simulink model "ode_engine_sim - preorg backup"  (R2022a)
settings: Solver=VariableStepAuto  StartTime=0.0  StopTime=10.0  RelTol=1e-3
model workspace (MAT data in the model file):
  A_inj = 1
  A_throat = 1
  C_d = 0.7
  L = 1
  L_grain = 1
  TCrit = 309.57
  V_tank = 1
  a = 1
  m_reg = 1
  n = 1
  rhoCrit = 452
  rho_f = 1
settings Model: Creator=Artem Sotnikov  LastModifiedBy=Artem Sotnikov

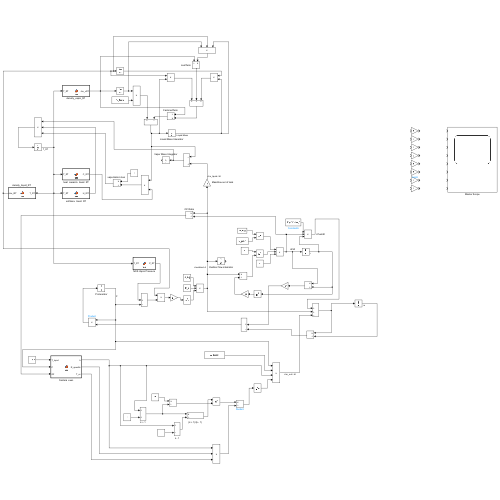
[thumbnail: Simulink's stored preview of the top-level diagram]
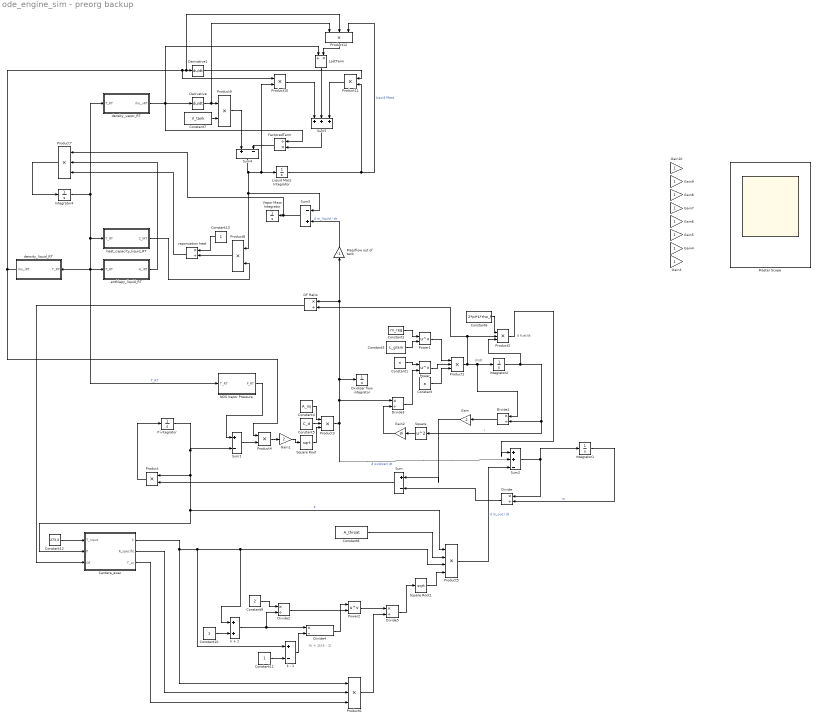
== system ode_engine_sim - preorg backup ==
  note: (k + 1)/(k - 1)
  note: d fuel/dt
  note: dr/dt
  Cantera_exec : MATLAB Function  TreatAsAtomicUnit=on
  Constant : Constant  Value=a
  Constant1 : Constant  Value=n
  Constant10 : Constant
  Constant11 : Constant
  Constant12 : Constant  Value=273.3
  Constant13 : Constant
  Constant2 : Constant  Value=m_reg
  Constant3 : Constant  Value=L_grain
  Constant4 : Constant  Value=A_inj
  Constant5 : Constant  Value=C_d
  Constant6 : Constant  Value=2*pi*L*rho_f
  Constant7 : Constant  Value=V_tank
  Constant8 : Constant  Value=A_throat
  Constant9 : Constant  Value=2
  Derivative : Derivative
  Derivative1 : Derivative
  Divide{,1..5} (6 alike) : Product  Inputs=*/
  FactoredTerm : Product  Inputs=/*
  Gain : Gain  Gain=2
  Gain1 : Gain  Gain=2
  Gain{3..10} (8 alike) : Gain
  Gain2 : Gain  Gain=pi
  Integrator1 : Integrator
  Integrator2 : Integrator
  Integrator4 : Integrator
  LastTerm : Product  Inputs=/*
  Liquid Mass Integrator : Integrator
  Massflow out of tank : Gain  Gain=-1
  Master Scope : Scope  NumInputPorts=8
  NOS Vapor Pressure : MATLAB Function  TreatAsAtomicUnit=on
  OF Ratio : Product  Inputs=*/
  Oxidizer flow integrator : Integrator
  P integrator : Integrator
  Power : Math  Operator=pow
  Power1 : Math  Operator=pow
  Power2 : Math  Operator=pow
  Product{,4,8..11} (6 alike) : Product
  Product{1..3,6..7,12} (6 alike) : Product  Inputs=3
  Product5 : Product  Inputs=4
  Square : Math  Operator=square
  Square Root : Sqrt
  Square Root1 : Sqrt
  Sum : Sum  Inputs=|+-
  Sum1 : Sum  Inputs=|+-
  Sum2 : Sum  Inputs=|++-
  Sum3 : Sum  Inputs=-+
  Sum4 : Sum  Inputs=+-
  Sum5 : Sum  Inputs=+++
  Vapor Mass Integrator : Integrator
  "density_liquid_RT " : MATLAB Function  TreatAsAtomicUnit=on
  density_vapor_RT : MATLAB Function  TreatAsAtomicUnit=on
  enthlapy_liquid_RT : MATLAB Function  TreatAsAtomicUnit=on
  heat_capacity_liquid_RT : MATLAB Function  TreatAsAtomicUnit=on
  k + 1 : Sum
  k - 1 : Sum  Inputs=+-
  vaporization heat : Product  Inputs=*/
  wires:
  P integrator/1 -> Sum1/2, Product/1, Product5/1, Cantera_exec/2(P)  "P"
  Sum/1 -> Product/2
  Integrator1/1 -> Divide/2  "m"
  Product/1 -> P integrator/1
  Sum2/1 -> Integrator1/1, Divide/1
  Divide/1 -> Sum/2
  Product1/1 -> Integrator2/1, Divide1/1, Product2/2, OF Ratio/2
  Integrator2/1 -> Product2/3, Divide1/2, Square/1  "r"
  Divide1/1 -> Gain/1
  Gain/1 -> Sum/1
  Power/1 -> Product1/2
  Power1/1 -> Product1/1
  Constant/1 -> Product1/3
  Constant1/1 -> Power/1
  Constant2/1 -> Power1/1
  Constant3/1 -> Power1/2
  Divide3/1 -> Power/2
  Constant5/1 -> Product3/2
  Constant4/1 -> Product3/1
  Square Root/1 -> Product3/3
  Product3/1 -> Sum2/2, Divide3/1, Massflow out of tank/1, OF Ratio/1, Oxidizer flow integrator/1  "d oxidizer/ dt"
  Gain1/1 -> Square Root/1
  NOS Vapor Pressure/1(P_RT) -> Sum1/1
  Product4/1 -> Gain1/1
  Sum1/1 -> Product4/2
  "density_liquid_RT "/1(rho_lRT) -> Product10/1, Product12/2, Derivative1/1, Product4/1
  Square/1 -> Gain2/1
  Gain2/1 -> Divide3/2
  Product2/1 -> Sum2/1
  Constant6/1 -> Product2/1
  Product5/1 -> Sum2/3  "d m_out / dt"
  Square Root1/1 -> Product5/4
  Constant8/1 -> Product5/2
  Cantera_exec/1(k) -> Product6/1, Product5/3, k + 1/1, k - 1/1
  Constant9/1 -> Divide2/1
  Constant10/1 -> k + 1/2
  k + 1/1 -> Divide4/1, Divide2/2
  k - 1/1 -> Divide4/2
  Constant11/1 -> k - 1/2
  Divide4/1 -> Power2/1
  Divide2/1 -> Power2/2
  Product6/1 -> Divide5/2
  Power2/1 -> Divide5/1
  Cantera_exec/2(R_specific) -> Product6/2
  Constant12/1 -> Cantera_exec/1(T_input)
  OF Ratio/1 -> Cantera_exec/3(OF)
  Cantera_exec/3(T_cc) -> Product6/3
  Divide5/1 -> Square Root1/1
  Integrator4/1 -> NOS Vapor Pressure/1(T_RT), "density_liquid_RT "/1(T_RT), enthlapy_liquid_RT/1(T_RT), heat_capacity_liquid_RT/1(T_RT), density_vapor_RT/1(T_RT)  "T_RT"
  Product7/1 -> Integrator4/1
  enthlapy_liquid_RT/1(H_lRT) -> Product7/2
  Constant13/1 -> vaporization heat/1
  Product8/1 -> vaporization heat/2
  heat_capacity_liquid_RT/1(C_lRT) -> Product8/2
  vaporization heat/1 -> Product7/3
  Massflow out of tank/1 -> Sum3/2  "d m_liquid / dt"
  Sum3/1 -> Product7/1, Vapor Mass Integrator/1
  Sum4/1 -> Product8/1, Sum3/1, Liquid Mass Integrator/1, Product10/2
  Liquid Mass Integrator/1 -> Product11/2, Product12/3  "Liquid Mass"
  Product9/1 -> Sum4/1
  density_vapor_RT/1(rho_vRT) -> Derivative/1, FactoredTerm/1, LastTerm/1
  Derivative/1 -> Product9/1, Product12/1
  Constant7/1 -> Product9/2
  Product10/1 -> Sum5/1
  FactoredTerm/1 -> Sum4/2
  Sum5/1 -> FactoredTerm/2
  Derivative1/1 -> Product11/1
  Product11/1 -> Sum5/3
  Product12/1 -> LastTerm/2
  LastTerm/1 -> Sum5/2

== matlab function ode_engine_sim - preorg backup/NOS Vapor Pressure ==
  data: T_RT input; P_RT output
function P_RT = fcn(T_RT)

p = [1.0, 1.5, 2.5, 5.0];
b = [-6.71893, 1.35966, -1.3779, -4.051];

Tr = T_RT / TCrit;
Tr_minus_one_vP = 1.0 - Tr;
acc_vP = 0.0;

for idx = [1,2,3,4]
    acc_vP = acc_vP + b(idx) * Tr_minus_one_vP^p(idx);
end

P_RT = PCrit * e^((acc_vP / Tr));

== matlab function ode_engine_sim - preorg backup/Cantera_exec ==
  data: k output; R_specific output; T_input input; T_cc output; P input; OF input
function [k, R_specific, T_cc] = fcn(T_input, P, OF)

ThermoModel.TPY = [T_input, P, OF];

ThermoModel.equilibrate('HP')


T_cc = ThermoModel.T;
k = ThermoModel.k;
R_specific = 8314 / ThermoModel.mean_molecular_weight;

== matlab function ode_engine_sim - preorg backup/heat_capacity_liquid_RT ==
  data: T_RT input; C_lRT output
function C_lRT = fcn(T_RT)

b = [2.49973, 0.023454, -3.80136, 13.0945, -14.518];

Tr_C = T_RT / tCrit;
Tr_C_minus_one = 1.0 - Tr_C;
acc = 1.0 + b(1) / Tr_minus_one;


for idx = [1,2,3,4]
    acc = acc + b(idx) * Tr_C_minus_one^idx;
end

result = b(0) * acc * 1000.0 # convert from KJ to J */

C_lRT = T_RT;

== matlab function ode_engine_sim - preorg backup/enthlapy_liquid_RT ==
  data: T_RT input; H_lRT output
function H_lRT = fcn(T_RT)
bL = [-200.0, 116.043, -917.225, 794.779, -589.587];
bV = [-200.0, 440.055, -459.701, 434.081, -485.338];

Tr_H = T_RT / TCrit;
Tr_H_minus_one = 1.0 - Tr_H;
acc_L = bL(0);
acc_V = bV(0);


for idx = [1,2,3,4,5]
    acc_L = acc_L + bL(idx) * Tr_H_minus_one^(idx / 3.0); 
    acc_V = acc_V + bV(idx) * Tr_H_minus_one^(idx / 3.0); 
end

result = (acc_V - acc_L) * 1000.0;

H_lRT = result;

== matlab function ode_engine_sim - preorg backup/density_liquid_RT  ==
  data: T_RT input; rho_lRT output
function rho_lRT = fcn(T_RT)

b = [1.72328, -0.8395, 0.5106, -0.10412];

Tr_l = T_RT / TCrit;
Tr_l_minus_one = 1.0 - Tr_l;
acc_l = 0.0;

for idx = [1,2,3,4]
    acc_l = acc_l + b(idx)* Tr_l_minus_one^(idx/3.0);
end

rho_lRT = rhoCrit * e^acc_l;

== matlab function ode_engine_sim - preorg backup/density_vapor_RT ==
  data: T_RT input; rho_vRT output
function rho_vRT = fcn(T_RT)

b = [-1.009, -6.28792, 7.50332, -7.90463, 0.629427];

Tr_v = T_RT / TCrit;
Tr_v_minus_one = 1.0 - Tr_v;
acc_v = 0.0;

for idx = [1,2,3,4,5]
    acc_v = acc_v + b(idx) * Tr_v_minus_one^(idx/3.0);
end


rho_vRT = rhoCrit * e^acc_v;
